simulink model "untitled"  (R2023b)
settings: Solver=VariableStepAuto  StartTime=0.0  StopTime=10.0  RelTol=1e-3
undefined symbols (not defined in the file): A, B, C, D, k1, k2
settings Model: Creator=haoyuan  LastModifiedBy=haoyuan

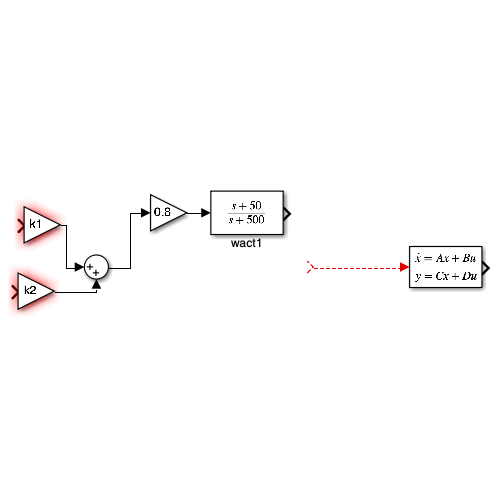
[thumbnail: Simulink's stored preview of the top-level diagram]
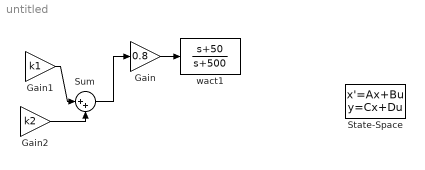
== system untitled ==
  Gain : Gain  Gain=0.8
  Gain1 : Gain  Gain=k1
  Gain2 : Gain  Gain=k2
  State-Space : StateSpace  A=A  B=B  C=C  D=D  InitialCondition=0
  Sum : Sum  Inputs=|++
  wact1 : TransferFcn  Numerator=[1 50]  Denominator=[1 500]
  wires:
  ? -> State-Space/1
  Gain1/1 -> Sum/1
  Sum/1 -> Gain/1
  Gain2/1 -> Sum/2
  Gain/1 -> wact1/1
